simulink model "Astar"  (R2018b)
settings: Solver=FixedStepAuto  StartTime=0.0  StopTime=inf  FixedStep=0.05  RelTol=1e-3
model workspace (MAT data in the model file):
  SL_ROS_VariableLengthArrays_MaxSizes.CommonInfo.ArrayTruncateAction = 'EmitWarning'
  SL_ROS_VariableLengthArrays_MaxSizes.MsgTypeMap = containers.Map
  SL_ROS_VariableLengthArrays_MaxSizes.MsgTypeMap.serialization.keys = {'sensor_msgs/LaserScan'}
  SL_ROS_VariableLengthArrays_MaxSizes.MsgTypeMap.serialization.values{1}(1).PropertyName = 'Intensities'
  SL_ROS_VariableLengthArrays_MaxSizes.MsgTypeMap.serialization.values{1}(1).DataType = 'single'
  SL_ROS_VariableLengthArrays_MaxSizes.MsgTypeMap.serialization.values{1}(1).MaxLength = 360
  SL_ROS_VariableLengthArrays_MaxSizes.MsgTypeMap.serialization.values{1}(2).PropertyName = 'Ranges'
  SL_ROS_VariableLengthArrays_MaxSizes.MsgTypeMap.serialization.values{1}(2).DataType = 'single'
  SL_ROS_VariableLengthArrays_MaxSizes.MsgTypeMap.serialization.values{1}(2).MaxLength = 360
  SL_ROS_VariableLengthArrays_MaxSizes.MsgTypeMap.serialization.uniformity = 0
  SL_ROS_VariableLengthArrays_MaxSizes.MsgTypeMap.serialization.keyType = 'char'
  SL_ROS_VariableLengthArrays_MaxSizes.MsgTypeMap.serialization.valueType = 'any'
undefined symbols (not defined in the file): Angular, Linear
libraries: robotlib x6, simulink x1
settings Model: Creator=Kim Hyup  LastModifiedBy=Kim Hyup
settings OptimizationCC: EnhancedBackFolding=on  PassReuseOutputArgsAs=Individual arguments  MaxStackSize=64  OptimizeBlockOrder=speed  DifferentSizesBufferReuse=on  OptimizationCustomize=off
settings DebuggingCC: ParameterTunabilityLossMsg=error
settings HardwareCC: ProdBitPerPointer=32  ProdBitPerSizeT=32  ProdBitPerPtrDiffT=32  ProdLargestAtomicFloat=None  ProdIntDivRoundTo=Undefined  ProdEndianess=Unspecified  ProdWordSize=32  ProdHWDeviceType=Generic->Unspecified (assume 32-bit Generic)  UseEmbeddedCoderFeatures=off
settings SFSimCC: MATLABDynamicMemAlloc=off
settings RTWCC: SystemTargetFile=ert.tlc  HardwareBoard=Robot Operating System (ROS)  TLCOptions="-aInlineSetEventsForThisBaseRateFcn=TLC_FALSE -aSuppressMultiTaskScheduler=TLC_FALSE  -aRateBasedStepFcn=0"  TemplateMakefile=ert_default_tmf  GenerateReport=on  Toolchain=Catkin  IncludeHyperlinkInReport=on  LaunchReport=on  TargetLang=C++  GenerateTraceInfo=on  GenerateTraceReport=on  GenerateTraceReportSl=on  GenerateTraceReportSf=on  GenerateTraceReportEml=on
settings CodeAppCC: ForceParamTrailComments=on  IgnoreCustomStorageClasses=off  OperatorAnnotations=on  SimulinkDataObjDesc=on  SFDataObjDesc=on  InsertBlockDesc=on
settings ERTTargetCC: SupportNonInlinedSFcns=on

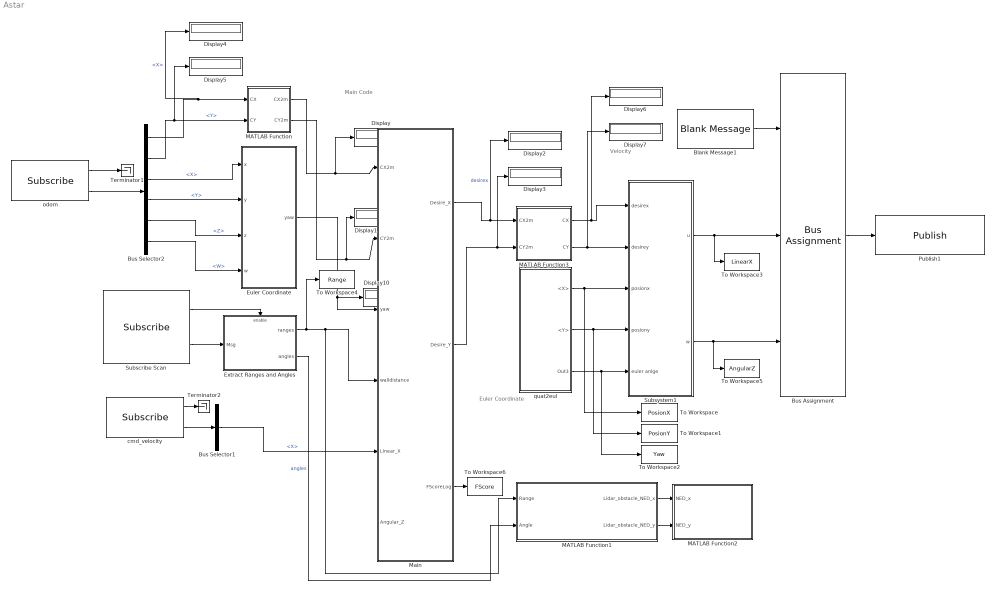
== system Astar ==
  note: Main Code
  note: Euler Coordinate
  note: Velocity
  Blank Message1 : robotlib/Blank Message  messageClass=Message  entityType=geometry_msgs/Twist  messageType=geometry_msgs/Twist  SampleTime=inf
      settings: SourceProductBaseCode=RO
  Bus Assignment : BusAssignment  AssignedSignals=Linear.X,Angular.Z
  Bus Selector1 : BusSelector  OutputSignals=Linear.X
  Bus Selector2 : BusSelector  OutputSignals=Pose.Pose.Position.X,Pose.Pose.Position.Y,Pose.Pose.Orientation.X,Pose.Pose.Orientation.Y,Pose.Pose.Orientation.Z,Pose.Pose.Orientation.W
  Display{,1..7,10} (9 alike) : Display
  Euler Coordinate : MATLAB Function  TreatAsAtomicUnit=on
  Extract Ranges and Angles : Subsystem  TreatAsAtomicUnit=on
  MATLAB Function : MATLAB Function  TreatAsAtomicUnit=on
  MATLAB Function1 : MATLAB Function  TreatAsAtomicUnit=on
  MATLAB Function2 : MATLAB Function  TreatAsAtomicUnit=on
  MATLAB Function3 : MATLAB Function  TreatAsAtomicUnit=on
  Main : MATLAB Function  TreatAsAtomicUnit=on
  Publish1 : robotlib/Publish  topicSource=Select from ROS network  topic=/cmd_vel  messageType=geometry_msgs/Twist  messageQueueLength=1
      settings: SourceProductBaseCode=RO
  Subscribe Scan : robotlib/Subscribe  topicSource=Select from ROS network  topic=/scan  messageType=sensor_msgs/LaserScan  sampleTime=-1  messageQueueLength=1
      settings: SourceProductBaseCode=RO
  Subsystem1 : Subsystem
  Terminator1 : Terminator
  Terminator2 : Terminator
  To Workspace : ToWorkspace  VariableName=PosionX  SaveFormat=Timeseries  SampleTime=-1
  To Workspace1 : ToWorkspace  VariableName=PosionY  SaveFormat=Timeseries  SampleTime=-1
  To Workspace2 : ToWorkspace  VariableName=Yaw  SaveFormat=Timeseries  SampleTime=-1
  To Workspace3 : ToWorkspace  VariableName=LinearX  SaveFormat=Timeseries  SampleTime=-1
  To Workspace4 : ToWorkspace  VariableName=Range  SaveFormat=Timeseries  SampleTime=-1
  To Workspace5 : ToWorkspace  VariableName=AngularZ  SaveFormat=Timeseries  SampleTime=-1
  To Workspace6 : ToWorkspace  VariableName=FScore  SaveFormat=Timeseries  SampleTime=-1
  cmd_velocity : robotlib/Subscribe  topicSource=Select from ROS network  topic=/cmd_vel  messageType=geometry_msgs/Twist  sampleTime=-1  messageQueueLength=1
      settings: SourceProductBaseCode=RO
  odom : robotlib/Subscribe  topicSource=Select from ROS network  topic=/odom  messageType=nav_msgs/Odometry  sampleTime=-1  messageQueueLength=1
      settings: SourceProductBaseCode=RO
  quat2eul : Subsystem
  wires:
  cmd_velocity/2 -> Bus Selector1/1
  odom/1 -> Terminator1/1
  odom/2 -> Bus Selector2/1
  cmd_velocity/1 -> Terminator2/1
  Bus Selector2/5 -> Euler Coordinate/3(z)  "<Z>"
  Bus Selector2/6 -> Euler Coordinate/4(w)  "<W>"
  Bus Selector2/4 -> Euler Coordinate/2(y)  "<Y>"
  Bus Selector2/3 -> Euler Coordinate/1(x)  "<X>"
  Subscribe Scan/1 -> Extract Ranges and Angles/Enable
  Subscribe Scan/2 -> Extract Ranges and Angles/1(Msg)
  Euler Coordinate/1(yaw) -> Display10/1, Main/3(yaw)
  Bus Selector1/1 -> Main/5(Linear_X)  "<X>"
  MATLAB Function1/1(Lidar_obstacle_NED_x) -> MATLAB Function2/1(NED_x)
  MATLAB Function1/2(Lidar_obstacle_NED_y) -> MATLAB Function2/2(NED_y)
  Bus Selector2/1 -> Display4/1, MATLAB Function/1(CX)  "<X>"
  Bus Selector2/2 -> Display5/1, MATLAB Function/2(CY)  "<Y>"
  MATLAB Function/2(CY2m) -> Display1/1, Main/2(CY2m)
  MATLAB Function/1(CX2m) -> Display/1, Main/1(CX2m)
  Extract Ranges and Angles/2(angles) -> MATLAB Function1/2(Angle)  "angles"
  Main/1(Desire_X) -> Display2/1, MATLAB Function3/1(CX2m)  "desirex"
  Main/2(Desire_Y) -> Display3/1, MATLAB Function3/2(CY2m)
  MATLAB Function3/1(CX) -> Display6/1, Subsystem1/1(desirex)
  MATLAB Function3/2(CY) -> Display7/1, Subsystem1/2(desirey)
  Extract Ranges and Angles/1(ranges) -> To Workspace4/1, MATLAB Function1/1(Range), Main/4(walldistance)
  quat2eul/1(<X>) -> To Workspace/1, Subsystem1/3(posionx)
  Subsystem1/2(w) -> To Workspace5/1, Bus Assignment/3
  Subsystem1/1(u) -> To Workspace3/1, Bus Assignment/2
  Blank Message1/1 -> Bus Assignment/1
  quat2eul/2(<Y>) -> To Workspace1/1, Subsystem1/4(posiony)
  quat2eul/3(Out3) -> To Workspace2/1, Subsystem1/5(euler anlge)
  Bus Assignment/1 -> Publish1/1
  Main/3(FScoreLog) -> To Workspace6/1

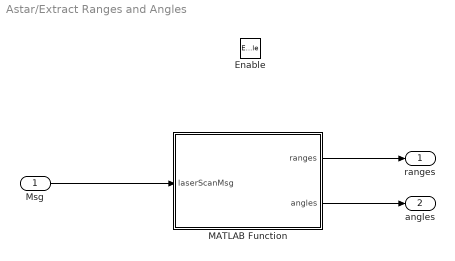
== system Astar/Extract Ranges and Angles ==
  Msg : Inport
  Enable : EnablePort
  MATLAB Function : MATLAB Function  TreatAsAtomicUnit=on
  ranges : Outport
  angles : Outport  Port=2
  wires:
  MATLAB Function/2(angles) -> angles/1
  Msg/1 -> MATLAB Function/1(laserScanMsg)
  MATLAB Function/1(ranges) -> ranges/1

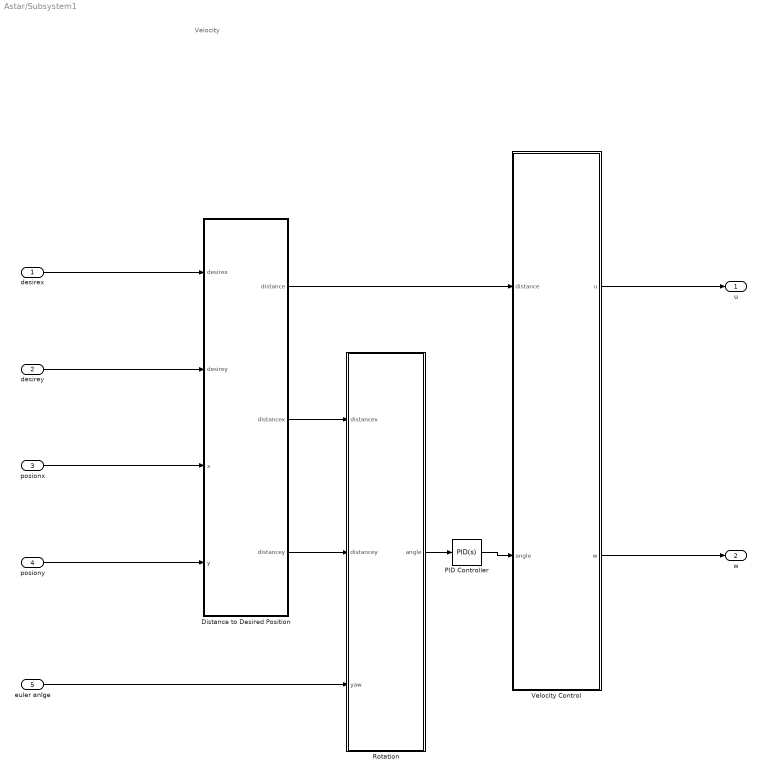
== system Astar/Subsystem1 ==
  note: Velocity
  desirex : Inport
  desirey : Inport  Port=2
  posionx : Inport  Port=3
  posiony : Inport  Port=4
  euler anlge : Inport  Port=5
  Distance to Desired Position : MATLAB Function  TreatAsAtomicUnit=on
  PID Controller : simulink/Continuous/PID Controller  Controller=PID  Form=Parallel  TimeDomain=Continuous-time  SampleTime=-1  IntegratorMethod=Forward Euler  FilterMethod=Forward Euler  ControllerParametersSource=internal  P=1.1  I=0  D=0  UseFilter=on  N=100  TunerSelectOption=Transfer Function Based (PID Tuner App)  InitialConditionSource=internal  InitialConditionForIntegrator=0  InitialConditionForFilter=0  DifferentiatorICPrevScaledInput=0  ExternalReset=none  TrackingMode=off  Kt=1  LimitOutput=off  UpperSaturationLimit=inf  LowerSaturationLimit=-inf  LinearizeAsGain=on  AntiWindupMode=none  Kb=1  POutMin=[]  POutMax=[]  IOutMin=[]  IOutMax=[]  DOutMin=[]  DOutMax=[]  NOutMin=[]  NOutMax=[]  SumOutMin=[]  SumOutMax=[]  SaturationOutMin=[]  SaturationOutMax=[]  PParamMin=[]  PParamMax=[]  IParamMin=[]  IParamMax=[]  DParamMin=[]  DParamMax=[]  NParamMin=[]  NParamMax=[]  KbParamMin=[]  KbParamMax=[]  KtParamMin=[]  KtParamMax=[]  KbOutMin=[]  KbOutMax=[]  KtOutMin=[]  KtOutMax=[]  IntegratorOutMin=[]  IntegratorOutMax=[]  FilterOutMin=[]  FilterOutMax=[]  SumI1OutMin=[]  SumI1OutMax=[]  SumI2OutMin=[]  SumI2OutMax=[]  SumI3OutMin=[]  SumI3OutMax=[]  SumI4OutMin=[]  SumI4OutMax=[]  SumDOutMin=[]  SumDOutMax=[]  DifferentiatorOutMin=[]  DifferentiatorOutMax=[]  FilterDiffOutCoefMin=[]  FilterDiffOutCoefMax=[]  ReciprocalOutMin=[]  ReciprocalOutMax=[]  SumDenOutMin=[]  SumDenOutMax=[]  SumNumOutMin=[]  SumNumOutMax=[]  DivideOutMin=[]  DivideOutMax=[]  IntegratorContinuousStateAttributes=''  IntegratorStateMustResolveToSignalObject=off  IntegratorRTWStateStorageClass=Auto  FilterContinuousStateAttributes=''  FilterStateMustResolveToSignalObject=off  FilterRTWStateStorageClass=Auto  ParallelPVariant=InternalParameters  IdealPVariant=Disabled  IVariant=InternalParameters  DVariant=InternalParameters  IntegratorVariant=Continuous  SatVariant=Disabled  AWVariant=Passthrough  PCopyVariant=Disabled  TRVariant=Disabled  FdbkBlocksVariant=Forward  IdealPFdbkVariant=Disabled  SatFdbkVariant=Disabled  DerivativeFilterVariant=ContFilter  NVariant=InternalParameters  NCopyVariant=Disabled  FilterICVariant=InternalICsFilter  IntegratorICVariant=InternalICs  ExternalResetVariant=Disabled  TRSumVariant=Passthrough  SumFdbkVariant=Disabled  SumVariant=Sum_PID
  Rotation : MATLAB Function  TreatAsAtomicUnit=on
  Velocity Control : MATLAB Function  TreatAsAtomicUnit=on
  u : Outport
  w : Outport  Port=2
  wires:
  desirex/1 -> Distance to Desired Position/1(desirex)
  Distance to Desired Position/3(distancey) -> Rotation/2(distancey)
  desirey/1 -> Distance to Desired Position/2(desirey)
  Distance to Desired Position/2(distancex) -> Rotation/1(distancex)
  Velocity Control/2(w) -> w/1
  posionx/1 -> Distance to Desired Position/3(x)
  euler anlge/1 -> Rotation/3(yaw)
  posiony/1 -> Distance to Desired Position/4(y)
  Rotation/1(angle) -> PID Controller/1
  PID Controller/1 -> Velocity Control/2(angle)
  Distance to Desired Position/1(distance) -> Velocity Control/1(distance)
  Velocity Control/1(u) -> u/1

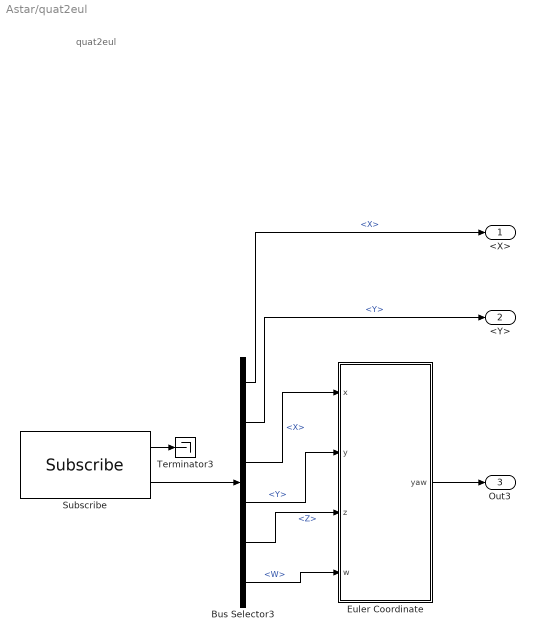
== system Astar/quat2eul ==
  note: quat2eul
  Bus Selector3 : BusSelector  OutputSignals=Pose.Pose.Position.X,Pose.Pose.Position.Y,Pose.Pose.Orientation.X,Pose.Pose.Orientation.Y,Pose.Pose.Orientation.Z,Pose.Pose.Orientation.W
  Euler Coordinate : MATLAB Function  TreatAsAtomicUnit=on
  Subscribe : robotlib/Subscribe  topicSource=Select from ROS network  topic=/odom  messageType=nav_msgs/Odometry  sampleTime=-1  messageQueueLength=1
      settings: SourceProductBaseCode=RO
  Terminator3 : Terminator
  <X> : Outport
  <Y> : Outport  Port=2
  Out3 : Outport  Port=3
  wires:
  Euler Coordinate/1(yaw) -> Out3/1
  Bus Selector3/5 -> Euler Coordinate/3(z)  "<Z>"
  Bus Selector3/6 -> Euler Coordinate/4(w)  "<W>"
  Subscribe/1 -> Terminator3/1
  Bus Selector3/3 -> Euler Coordinate/1(x)  "<X>"
  Subscribe/2 -> Bus Selector3/1
  Bus Selector3/4 -> Euler Coordinate/2(y)  "<Y>"
  Bus Selector3/2 -> <Y>/1  "<Y>"
  Bus Selector3/1 -> <X>/1  "<X>"

== matlab function Astar/quat2eul/Euler Coordinate ==
  data: x input; yaw output; y input; z input; w input
function yaw = quat2eul(x,y,z,w)

eul = quat2eul([w,x,y,z]);
yaw = eul(1);

end

== matlab function Astar/Main ==
  data: CX2m input; CY2m input; yaw input; Desire_X output size=1; walldistance input; Linear_X input; Desire_Y output size=1; Angular_Z input; FScoreLog output
function [Desire_X, Desire_Y, FScoreLog] = main(CX2m,CY2m,yaw, walldistance, Linear_X, Angular_Z)
%% 영속변수 설정, Define F(x)
persistent FScore GScore HScore ClosedMAT NodeXY Nodenumber Path Direction_X Direction_Y;

Look = 0.350; % 팬스의 길이 단위
RangeLimit = 0.230; % 장애물의 유무 기준 거리
Height = 4; % 미로 전체에서 x축에 필요한 팬스 갯수
Width = 4; % y축에 필요한 팬스 갯수
N = Height * Width;

if isempty(FScore)
    FScore = inf(Height+2,Width+2);
    GScore = inf(Height+2,Width+2);
    HScore = inf(Height+2,Width+2);
    ClosedMAT = zeros(Height+2,Width+2);
    NodeXY = inf(Height+2,Width+2);
    Nodenumber = 1;
    Path = inf(N,N);
    Direction_X = 0;
    Direction_Y = 0;
end

%% define Start, Goal (x,y)
Start = [2 2];
Goal = [5 5];
ClosedMAT(Start(1),Start(2)) = 1;

if (Linear_X <= 0.1) && (Angular_Z <=0.01)
    FScore = FScore + 0.1;

    %% define G(x) Search
    G_Search = [inf 1 inf;...
                  1 0   1;...
                inf 1 inf];
    GScore(Start(1),Start(2)) = 0;

    %% Define Heuristic
    for i=1:Height+2
        for j=1:Width+2
            HScore(i,j) = (abs(Goal(1)-i)+abs(Goal(2)-j));
        end
    end

    %% nodeXY 행렬에는 어떤 노드가 몇 번인지 나타낸다
    NodeXY(Start(1),Start(2)) = 1;
    %% 터틀봇이 바라보고 있는 방향에 따른 Up, Right, Down, Left 방향 설정
    Range1 = zeros(1,40); % UP
    Range2 = zeros(1,40); % Right
    Range3 = zeros(1,40); % Down
    Range4 = zeros(1,40); % Left
    
    if (yaw >= -0.2) && (yaw <= 0.2) % 고정좌표계 기준 '오른쪽'을 바라볼 때
        Range1(1:40) = walldistance(64:103);
        Range2(1:40) = walldistance(157:196);
        Range3(1:40) = walldistance(250:289);
        Range4(1:30) = walldistance(331:360);
        Range4(31:40) = walldistance(1:10);
    elseif (yaw >= (pi()/2)-0.2) && (yaw <= (pi()/2)+0.2) % '위쪽'을 바라볼 때
        Range1(1:40) = walldistance(157:196);
        Range2(1:40) = walldistance(250:289);
        Range3(1:30) = walldistance(331:360);
        Range3(31:40) = walldistance(1:10);
        Range4(1:40) = walldistance(64:103);
    elseif (yaw >= -(pi()/2)-0.2) && (yaw <= -(pi()/2)+0.2) % '아래쪽'을 바라볼 때
        Range1(1:30) = walldistance(331:360);
        Range1(31:40) = walldistance(1:10);
        Range2(1:40) = walldistance(64:103);
        Range3(1:40) = walldistance(157:196);
        Range4(1:40) = walldistance(250:289);
    elseif (yaw >= pi()-0.2) && (yaw <= -pi()+0.2) % '왼쪽'을 바라볼 때
        Range1(1:40) = walldistance(250:289);
        Range2(1:30) = walldistance(331:360);
        Range2(31:40) = walldistance(1:10);
        Range3(1:40) = walldistance(64:103);
        Range4(1:40) = walldistance(157:196);
    end


    %% 장애물 or 이미 방문한 노드 or 미로 범위를 벗어났는지 판별

    Search = ones(1,4);

    if max(Range1(1:40)) <= RangeLimit || ClosedMAT(CX2m,CY2m+1)==1 || CY2m+1 > Height % UP
        G_Search(1,2) = inf;
        Search(1) = 0;
    end

    if max(Range2(1:40)) <= RangeLimit || ClosedMAT(CX2m+1,CY2m)==1 || CX2m+1 > Width % Right
        G_Search(2,3) = inf;
        Search(2) = 0;
    end

    if max(Range3(1:40)) <= RangeLimit || ClosedMAT(CX2m,CY2m-1)==1 || CY2m-1 < 1 % Down
        G_Search(3,2) = inf;
        Search(3) = 0;
    end

    if max(Range4(1:40)) <= RangeLimit || ClosedMAT(CX2m-1,CY2m)==1 || CX2m-1 < 1 % Left
        G_Search(2,1) = inf;
        Search(4) = 0;
    end

    %%
    Prenodenumber = NodeXY(CX2m,CY2m);

    for i=1:4
        if Search(i) == 1
            if i == 1
                GScore(CX2m,CY2m+1) = GScore(CX2m,CY2m) + 0.1; % UP
                if NodeXY(CX2m,CY2m+1) == inf
                    Nodenumber = Nodenumber + 1;
                    NodeXY(CX2m,CY2m+1) = Nodenumber;
                end
            elseif i == 2 
                GScore(CX2m+1,CY2m) = GScore(CX2m,CY2m) + 0.1; % Right
                if NodeXY(CX2m+1,CY2m) == inf
                    Nodenumber = Nodenumber + 1;
                    NodeXY(CX2m+1,CY2m) = Nodenumber;
                end
            elseif i == 3
                GScore(CX2m,CY2m-1) = GScore(CX2m,CY2m) + 0.1; % Down
                if NodeXY(CX2m,CY2m-1) == inf
                    Nodenumber = Nodenumber + 1;
                    NodeXY(CX2m,CY2m-1) = Nodenumber;
                end
            else
                GScore(CX2m-1,CY2m) = GScore(CX2m,CY2m) + 0.1; % Left
                if NodeXY(CX2m-1,CY2m) == inf
                    Nodenumber = Nodenumber + 1;
                    NodeXY(CX2m-1,CY2m) = Nodenumber;
                end
            end
        end
    end

    %% 주변이 어떻게 탐색되었느냐에 따라
    if Prenodenumber ~= Nodenumber % 어느 한 방향이라도 탐색했다면
        FScore = GScore + HScore;
        ClosedMAT(CX2m,CY2m) = 1;
        FScore(ClosedMAT==1) = inf;
        MinFScore = min(min(FScore));
        [Min_x, Min_y] = find(FScore==MinFScore);

        Direction_X = Min_x(1,1);
        Direction_Y = Min_y(1,1);

        CurrentNode = NodeXY(CX2m,CY2m);
        NextNode = NodeXY(Direction_X,Direction_Y);
        Path(CurrentNode,NextNode) = 1;
    else % 4방향 모두 탐색 불가능이면 되돌아가야된다
        ClosedMAT(CX2m,CY2m) = 1;
        FScore(ClosedMAT==1) = inf;
        CurrentNode = NodeXY(CX2m,CY2m);
        NextNode = 1;
        for a=1:CurrentNode
            if Path(a,CurrentNode) == 1
                NextNode = a;
                break;
            end
        end
        Path(CurrentNode,NextNode) = inf;

        [Min_x, Min_y] = find(NodeXY==NextNode);

        Direction_X = Min_x(1,1);
        Direction_Y = Min_y(1,1);
    end
end
Desire_Y = Direction_X;
Desire_X = Direction_Y;
FScoreLog = FScore;
end

== matlab function Astar/Extract Ranges and Angles/MATLAB Function ==
  data: laserScanMsg input; ranges output size=360; angles output size=360
function [ranges, angles] = ExtractRangeData(laserScanMsg)
%#codegen

% Extract Range information
ranges = double(laserScanMsg.Ranges);

% Construct Angles vector using AngleMin and AngleIncrement from sensor
% reading.
angMin = double(laserScanMsg.AngleMin);
angIncrement = double(laserScanMsg.AngleIncrement);

numReadings = numel(ranges);
rawAngles = angMin + (0:numReadings-1)' * angIncrement;

% Wrap the angles to the (-pi,pi] interval.
angles = robotics.internal.wrapToPi(double(rawAngles));

== matlab function Astar/Subsystem1/Velocity Control ==
  data: distance input; u output; angle input; w output
function [u,w] = velocity(distance,angle)

if (angle <= 0.05) && (angle >= -0.05)
    if (distance >= 0.060)
        u = 0.2;
    else
        u = 0;
    end
elseif (angle <= 0.1) && (angle >= -0.1)
    u = 0.2;
else
    u = 0;
end

w = angle;

== matlab function Astar/Euler Coordinate ==
  data: x input; yaw output; y input; z input; w input
function yaw = quat2eul(x,y,z,w)

eul = quat2eul([w,x,y,z]);
yaw = eul(1);

end

== matlab function Astar/Subsystem1/Rotation ==
  data: distancex input; angle output; distancey input; yaw input
function angle = angle(distancex,distancey,yaw)

desireangle = atan2(distancey,distancex);
u = desireangle - yaw;
angle =  atan2(sin(u),cos(u));

== matlab function Astar/Subsystem1/Distance to Desired Position ==
  data: distance output; desirex input; distancex output; desirey input; x input; y input; distancey output
function [distance,distancex,distancey] = distance(desirex,desirey,x,y)

Height = 4;
Width = 4;
Look = 0.350;

for i=1:Height
    if (x >= (Look * (i - 1))-0.05) && (x <= (Look * (i + 1))+0.05)
        x = (Look * (i - 1));
    end
end
    
for i=1:Width
    if (y >= (Look * (i - 1))-0.05) && (y <= (Look * (i + 1))+0.05)
        y = (Look * (i - 1));
    end
end

distancex = desirex - x;
distancey = desirey - y;
distance = sqrt(distancex^2 + distancey^2);

== matlab function Astar/MATLAB Function1 ==
  data: Range input; Lidar_obstacle_NED_x output; Angle input; Lidar_obstacle_NED_y output
function [Lidar_obstacle_NED_x,Lidar_obstacle_NED_y] = Lidar(Range,Angle)

px = -Range .* cos(Angle);
py = Range .* sin(Angle);
Lidar_obstacle_NED_x = px';
Lidar_obstacle_NED_y = py';

end

== matlab function Astar/MATLAB Function2 ==
  data: NED_x input; NED_y input
function plotLaser(NED_x,NED_y)
coder.extrinsic('plot');

persistent p;
if isempty(p)
    p = plot(0,0,'.');
    set(gca,'xlim',[-4 4],'ylim',[-4 4],'YMinorGrid','on','XMinorGrid','on');
    % gca는 현재 Figure의 현재 좌표축 또는 차트를 반환합니다. 해당 좌표축 또는 차트는 
    % 일반적으로 가장 마지막에 생성되었거나 마우스로 클릭된 것입니다. title과 같은 그래픽스
    % 함수는 현재 좌표축 또는 차트를 대상으로 합니다. ax를 사용하여 좌표축 또는 차트의 속성에
    % 액세스하고 수정할 수 있습니다. 좌표축이나 차트가 없으면 gca는 카테시안 좌표축을 만듭니다.
    % 현재 gca = p;
end

if ishandle(p)
    % ishandle(H)는 H의 요소가 그래픽스이거나 Java® 객체 핸들인 경우 요소가 1인 배열을 반환하고,
    % 그렇지 않으면 요소가 0인 배열을 반환합니다.
    set(p,'XData',NED_y);
    set(p,'YData',NED_x);
    drawnow limitrate;
    % drawnow : Figure를 업데이트하고 보류 중인 콜백을 모두 처리
end

== matlab function Astar/MATLAB Function ==
  data: CX input; CX2m output; CY input; CY2m output
function [CX2m,CY2m] = carte2mat(CX,CY)
% 실제 위치를 행렬 위치로 바꾼다.

persistent Memory_X Memory_Y;

if isempty(Memory_X)
    Memory_X = 0;
    Memory_Y = 0;
end

Look = 0.350; % 팬스의 길이 단위
Height = 4; % 미로 전체에서 x축에 필요한 팬스 갯수
Width = 4; % y축에 필요한 팬스 갯수

n = 0;
for i=1:Height
    if (CX >= n-0.02) && (CX <= n+0.02)
        CX2m = i+1;
        Memory_X = i+1;
        break;
    end
    n = n + Look;
    CX2m = Memory_X;
end

n = 0;
for j=1:Width
    if (CY >= n-0.02) && (CY <= n+0.02)
        CY2m = j+1;
        Memory_Y = j+1;
        break;
    end
    n = n + Look;
    CY2m = Memory_Y;
end

== matlab function Astar/MATLAB Function3 ==
  data: CX2m input size=1; CX output; CY2m input size=1; CY output
function [CX,CY] = mat2carte(CX2m,CY2m)
% 행렬 위치를 실제 위치로 바꾼다.

Look = 0.350; % 팬스의 길이 단위

CX = (CX2m-2) * Look;
CY = (CY2m-2) * Look;
